simulink model "DrivetrainHevP4"  (R2023b)
settings: Solver=VariableStepAuto  StartTime=0.0  StopTime=inf  RelTol=1e-3  EnableMultiTasking=on
model workspace (MAT data in the model file):
  Aeff = Simulink.Parameter
  Aeff.Value = 0.0314159265359
  Aeff.DataType = 'double'
  Aeff.Complexity = 'real'
  Aeff.Dimensions = [1 1]
  Af = Simulink.Parameter
  Af.Value = 2.46
  Af.DataType = 'double'
  Af.Complexity = 'real'
  Af.Dimensions = [1 1]
  Bx = Simulink.Parameter
  Bx.Value = 10
  Bx.DataType = 'double'
  Bx.Complexity = 'real'
  Bx.Dimensions = [1 1]
  Cd = Simulink.Parameter
  Cd.Value = 0.25
  Cd.DataType = 'double'
  Cd.Complexity = 'real'
  Cd.Dimensions = [1 1]
  Cl = Simulink.Parameter
  Cl.Value = 0.1
  Cl.DataType = 'double'
  Cl.Complexity = 'real'
  Cl.Dimensions = [1 1]
  Cpm = Simulink.Parameter
  Cpm.Value = 0.1
  Cpm.DataType = 'double'
  Cpm.Complexity = 'real'
  Cpm.Dimensions = [1 1]
  Cx = Simulink.Parameter
  Cx.Value = 1.65
  Cx.DataType = 'double'
  Cx.Complexity = 'real'
  Cx.Dimensions = [1 1]
  Dx = Simulink.Parameter
  Dx.Value = 1
  Dx.DataType = 'double'
  Dx.Complexity = 'real'
  Dx.Dimensions = [1 1]
  Ex = Simulink.Parameter
  Ex.Value = 0.01
  Ex.DataType = 'double'
  Ex.Complexity = 'real'
  Ex.Dimensions = [1 1]
  FZMAX = Simulink.Parameter
  FZMAX.Value = 6570
  FZMAX.DataType = 'double'
  FZMAX.Complexity = 'real'
  FZMAX.Dimensions = [1 1]
  FZMIN = Simulink.Parameter
  FZMIN.Value = 0
  FZMIN.DataType = 'double'
  FZMIN.Complexity = 'real'
  FZMIN.Dimensions = [1 1]
  Fc = Simulink.Parameter
  Fc.Value = 500
  Fc.DataType = 'double'
  Fc.Complexity = 'real'
  Fc.Dimensions = [1 1]
  FsbF = Simulink.Parameter
  FsbF.Value = [-700000 -7000 -700 0 700 7000 700000]
  FsbF.DataType = 'double'
  FsbF.Complexity = 'real'
  FsbF.Dimensions = [1 7]
  FsbR = Simulink.Parameter
  FsbR.Value = [-700000 -7000 -700 0 700 7000 700000]
  FsbR.DataType = 'double'
  FsbR.Complexity = 'real'
  FsbR.Dimensions = [1 7]
  FskF = Simulink.Parameter
  FskF.Value = [-8928.57142857 -178.571428571 0 357.142857143 535.714285714 9285.71428571]
  FskF.DataType = 'double'
  FskF.Complexity = 'real'
  FskF.Dimensions = [1 6]
  FskR = Simulink.Parameter
  FskR.Value = [-5357.14285714 -107.142857143 0 214.285714286 321.428571429 5571.42857143]
  FskR.DataType = 'double'
  FskR.Complexity = 'real'
  FskR.Dimensions = [1 6]
  G = Simulink.Parameter
  G.Value = [0 1 2 3 4 5 6]
  G.DataType = 'double'
  G.Complexity = 'real'
  G.Dimensions = [1 7]
  G_o = Simulink.Parameter
  G_o.Value = 1
  G_o.DataType = 'double'
  G_o.Complexity = 'real'
  G_o.Dimensions = [1 1]
  Iyy = Simulink.Parameter
  Iyy.Value = 3000
  Iyy.DataType = 'double'
  Iyy.Complexity = 'real'
  Iyy.Dimensions = [1 1]
  Iyy_Whl = Simulink.Parameter
  Iyy_Whl.Value = 0.8
  Iyy_Whl.DataType = 'double'
  Iyy_Whl.Complexity = 'real'
  Iyy_Whl.Dimensions = [1 1]
  J = Simulink.Parameter
  J.Value = 0.01
  J.DataType = 'double'
  J.Complexity = 'real'
  J.Dimensions = [1 1]
  J1 = Simulink.Parameter
  J1.Value = 0.01
  J1.DataType = 'double'
  J1.Complexity = 'real'
  J1.Dimensions = [1 1]
  J2 = Simulink.Parameter
  J2.Value = 0.01
  J2.DataType = 'double'
  J2.Complexity = 'real'
  J2.Dimensions = [1 1]
  Jd = Simulink.Parameter
  Jd.Value = 0.01
  Jd.DataType = 'double'
  Jd.Complexity = 'real'
  Jd.Dimensions = [1 1]
  Ji = Simulink.Parameter
  Ji.Value = 0.2
  Ji.DataType = 'double'
  Ji.Complexity = 'real'
  Ji.Dimensions = [1 1]
  Jin = Simulink.Parameter
  Jin.Value = 0.05
  Jin.DataType = 'double'
  Jin.Complexity = 'real'
  Jin.Dimensions = [1 1]
  Jin_Cltch = Simulink.Parameter
  Jin_Cltch.Value = 0.2
  Jin_Cltch.DataType = 'double'
  Jin_Cltch.Complexity = 'real'
  Jin_Cltch.Dimensions = [1 1]
  Jin_Cltch2 = Simulink.Parameter
  Jin_Cltch2.Value = 0.01
  Jin_Cltch2.DataType = 'double'
  Jin_Cltch2.Complexity = 'real'
  Jin_Cltch2.Dimensions = [1 1]
  Jout = Simulink.Parameter
  Jout.Value = [0.009 0.01 0.01 0.01 0.01 0.01 0.01]
  Jout.DataType = 'double'
  Jout.Complexity = 'real'
  Jout.Dimensions = [1 7]
  Jout_Cltch = Simulink.Parameter
  Jout_Cltch.Value = 0.01
  Jout_Cltch.DataType = 'double'
  Jout_Cltch.Complexity = 'real'
  Jout_Cltch.Dimensions = [1 1]
  Jout_Cltch2 = Simulink.Parameter
  Jout_Cltch2.Value = 0.05
  Jout_Cltch2.DataType = 'double'
  Jout_Cltch2.Complexity = 'real'
  Jout_Cltch2.Dimensions = [1 1]
  Jt = Simulink.Parameter
  Jt.Value = 0.01
  Jt.DataType = 'double'
  Jt.Complexity = 'real'
  Jt.Dimensions = [1 1]
  Jw1 = Simulink.Parameter
  Jw1.Value = 0.01
  Jw1.DataType = 'double'
  Jw1.Complexity = 'real'
  Jw1.Dimensions = [1 1]
  Jw2 = Simulink.Parameter
  Jw2.Value = 0.01
  Jw2.DataType = 'double'
  Jw2.Complexity = 'real'
  Jw2.Dimensions = [1 1]
  K_c = Simulink.Parameter
  K_c.Value = 10000
  K_c.DataType = 'double'
  K_c.Complexity = 'real'
  K_c.Dimensions = [1 1]
  Lrel = Simulink.Parameter
  Lrel.Value = 0.15
  Lrel.DataType = 'double'
  Lrel.Complexity = 'real'
  Lrel.Dimensions = [1 1]
  Mass = Simulink.Parameter
  Mass.Value = 1623
  Mass.DataType = 'double'
  Mass.Complexity = 'real'
  Mass.Dimensions = [1 1]
  N = Simulink.Parameter
  N.Value = [1 4.212 2.637 1.8 1.386 1 0.772]
  N.DataType = 'double'
  N.Complexity = 'real'
  N.Dimensions = [1 7]
  NF = Simulink.Parameter
  NF.Value = 2
  NF.DataType = 'double'
  NF.Complexity = 'real'
  NF.Dimensions = [1 1]
  NR = Simulink.Parameter
  NR.Value = 2
  NR.DataType = 'double'
  NR.Complexity = 'real'
  NR.Dimensions = [1 1]
  N_P4 = Simulink.Parameter
  N_P4.Value = 4.1
  N_P4.DataType = 'double'
  N_P4.Complexity = 'real'
  N_P4.Dimensions = [1 1]
  Ndiff = Simulink.Parameter
  Ndiff.Value = 3.32
  Ndiff.DataType = 'double'
  Ndiff.Complexity = 'real'
  Ndiff.Dimensions = [1 1]
  Ndiff_P4 = Simulink.Parameter
  Ndiff_P4.Value = 4.1
  Ndiff_P4.DataType = 'double'
  Ndiff_P4.Complexity = 'real'
  Ndiff_P4.Dimensions = [1 1]
  Ndisk = Simulink.Parameter
  Ndisk.Value = 1
  Ndisk.DataType = 'double'
  Ndisk.Complexity = 'real'
  Ndisk.Dimensions = [1 1]
  Ndisks = Simulink.Parameter
  Ndisks.Value = 4
  Ndisks.DataType = 'double'
  Ndisks.Complexity = 'real'
  Ndisks.Dimensions = [1 1]
  Pabs = Simulink.Parameter
  Pabs.Value = 101325
  Pabs.DataType = 'double'
  Pabs.Complexity = 'real'
  Pabs.Dimensions = [1 1]
  Press = Simulink.Parameter
  Press.Value = 7000000
  Press.DataType = 'double'
  Press.Complexity = 'real'
  Press.Dimensions = [1 1]
  Re = Simulink.Parameter
  Re.Value = 0.327
  Re.DataType = 'double'
  Re.Complexity = 'real'
  Re.Dimensions = [1 1]
  Reff = Simulink.Parameter
  Reff.Value = 0.11
  Reff.DataType = 'double'
  Reff.Complexity = 'real'
  Reff.Dimensions = [1 1]
  Reff_LSD = Simulink.Parameter
  Reff_LSD.Value = 0.2
  Reff_LSD.DataType = 'double'
  Reff_LSD.Complexity = 'real'
  Reff_LSD.Dimensions = [1 1]
  Rm = Simulink.Parameter
  Rm.Value = 0.15
  Rm.DataType = 'double'
  Rm.Complexity = 'real'
  Rm.Dimensions = [1 1]
  T = Simulink.Parameter
  T.Value = 300
  T.DataType = 'double'
  T.Complexity = 'real'
  T.Dimensions = [1 1]
  Temp_bpts = Simulink.Parameter
  Temp_bpts.Value = [313 358]
  Temp_bpts.DataType = 'double'
  Temp_bpts.Complexity = 'real'
  Temp_bpts.Dimensions = [1 2]
  Trq_bpts = Simulink.Parameter
  Trq_bpts.Value = [25 50 75 100 150 200 250]
  Trq_bpts.DataType = 'double'
  Trq_bpts.Complexity = 'real'
  Trq_bpts.Dimensions = [1 7]
  UNLOADED_RADIUS = Simulink.Parameter
  UNLOADED_RADIUS.Value = 0.336
  UNLOADED_RADIUS.DataType = 'double'
  UNLOADED_RADIUS.Complexity = 'real'
  UNLOADED_RADIUS.Dimensions = [1 1]
  VXLOW = Simulink.Parameter
  VXLOW.Value = 2
  VXLOW.DataType = 'double'
  VXLOW.Complexity = 'real'
  VXLOW.Dimensions = [1 1]
  aMy = Simulink.Parameter
  aMy.Value = 0.01
  aMy.DataType = 'double'
  aMy.Complexity = 'real'
  aMy.Dimensions = [1 1]
  a_CG = Simulink.Parameter
  a_CG.Value = 1.09
  a_CG.DataType = 'double'
  a_CG.Complexity = 'real'
  a_CG.Dimensions = [1 1]
  alphaMy = Simulink.Parameter
  alphaMy.Value = 0
  alphaMy.DataType = 'double'
  alphaMy.Complexity = 'real'
  alphaMy.Dimensions = [1 1]
  b = Simulink.Parameter
  b.Value = 400
  b.DataType = 'auto'
  b.Complexity = 'real'
  b.Dimensions = [1 1]
  b1 = Simulink.Parameter
  b1.Value = 100
  b1.DataType = 'double'
  b1.Complexity = 'real'
  b1.Dimensions = [1 1]
  b1_g = Simulink.Parameter
  b1_g.Value = 0.001
  b1_g.DataType = 'double'
  b1_g.Complexity = 'real'
  b1_g.Dimensions = [1 1]
  b2 = Simulink.Parameter
  b2.Value = 100
  b2.DataType = 'double'
  b2.Complexity = 'real'
  b2.Dimensions = [1 1]
  b2_g = Simulink.Parameter
  b2_g.Value = 0.001
  b2_g.DataType = 'double'
  b2_g.Complexity = 'real'
  b2_g.Dimensions = [1 1]
  bMy = Simulink.Parameter
  bMy.Value = 0
  bMy.DataType = 'double'
  bMy.Complexity = 'real'
  bMy.Dimensions = [1 1]
  b_CG = Simulink.Parameter
  b_CG.Value = 1.7
  b_CG.DataType = 'double'
  b_CG.Complexity = 'real'
  b_CG.Dimensions = [1 1]
  b_J = Simulink.Parameter
  b_J.Value = 0.001
  b_J.DataType = 'double'
  b_J.Complexity = 'real'
  b_J.Dimensions = [1 1]
  bd = Simulink.Parameter
  bd.Value = 0.001
  bd.DataType = 'double'
  bd.Complexity = 'real'
  bd.Dimensions = [1 1]
  betaMy = Simulink.Parameter
  betaMy.Value = 1
  betaMy.DataType = 'double'
  betaMy.Complexity = 'real'
  betaMy.Dimensions = [1 1]
  bi = Simulink.Parameter
  bi.Value = 0.001
  bi.DataType = 'double'
  bi.Complexity = 'real'
  bi.Dimensions = [1 1]
  bin = Simulink.Parameter
  bin.Value = 0.003
  bin.DataType = 'double'
  bin.Complexity = 'real'
  bin.Dimensions = [1 1]
  bin_Cltch = Simulink.Parameter
  bin_Cltch.Value = 0.003
  bin_Cltch.DataType = 'double'
  bin_Cltch.Complexity = 'real'
  bin_Cltch.Dimensions = [1 1]
  bout = Simulink.Parameter
  bout.Value = [0.003 0.003 0.003 0.003 0.003 0.003 0.003]
  bout.DataType = 'double'
  bout.Complexity = 'real'
  bout.Dimensions = [1 7]
  bout_Cltch = Simulink.Parameter
  bout_Cltch.Value = 0.003
  bout_Cltch.DataType = 'double'
  bout_Cltch.Complexity = 'real'
  bout_Cltch.Dimensions = [1 1]
  br = Simulink.Parameter
  br.Value = 0.001
  br.DataType = 'double'
  br.Complexity = 'real'
  br.Dimensions = [1 1]
  bt = Simulink.Parameter
  bt.Value = 0.001
  bt.DataType = 'double'
  bt.Complexity = 'real'
  bt.Dimensions = [1 1]
  bw1 = Simulink.Parameter
  bw1.Value = 0.001
  bw1.DataType = 'double'
  bw1.Complexity = 'real'
  bw1.Dimensions = [1 1]
  bw2 = Simulink.Parameter
  bw2.Value = 0.001
  bw2.DataType = 'double'
  bw2.Complexity = 'real'
  bw2.Dimensions = [1 1]
  cMy = Simulink.Parameter
  cMy.Value = 0
  cMy.DataType = 'double'
  cMy.Complexity = 'real'
  cMy.Dimensions = [1 1]
  disk_abore = Simulink.Parameter
  disk_abore.Value = 0.05
  disk_abore.DataType = 'double'
  disk_abore.Complexity = 'real'
  disk_abore.Dimensions = [1 1]
  domega_o = Simulink.Parameter
  domega_o.Value = 0
  domega_o.DataType = 'double'
  domega_o.Complexity = 'real'
  domega_o.Dimensions = [1 1]
  dw = Simulink.Parameter
  dw.Value = [0 10 20 40 60 80 100]
  dw.DataType = 'double'
  dw.Complexity = 'real'
  dw.Dimensions = [1 7]
  dzdotsF = Simulink.Parameter
  dzdotsF.Value = [-10 -1 -0.1 0 0.1 1 10]
  dzdotsF.DataType = 'double'
  dzdotsF.Complexity = 'real'
  dzdotsF.Dimensions = [1 7]
  dzdotsR = Simulink.Parameter
  dzdotsR.Value = [-10 -1 -0.1 0 0.1 1 10]
  dzdotsR.DataType = 'double'
  dzdotsR.Complexity = 'real'
  dzdotsR.Dimensions = [1 7]
  dzsF = Simulink.Parameter
  dzsF.Value = [-0.005 -0.0001 0 0.2 0.2001 0.2051]
  dzsF.DataType = 'double'
  dzsF.Complexity = 'real'
  dzsF.Dimensions = [1 6]
  dzsR = Simulink.Parameter
  dzsR.Value = [-0.005 -0.0001 0 0.2 0.2001 0.2051]
  dzsR.DataType = 'double'
  dzsR.Complexity = 'real'
  dzsR.Dimensions = [1 6]
  eta = Simulink.Parameter
  eta.Value = [0.95 0.95 0.95 0.95 0.95 0.95 0.95]
  eta.DataType = 'double'
  eta.Complexity = 'real'
  eta.Dimensions = [1 7]
  eta_diff = Simulink.Parameter
  eta_diff.Value = 0.98
  eta_diff.DataType = 'double'
  eta_diff.Complexity = 'real'
  eta_diff.Dimensions = [1 1]
  eta_tbl = Simulink.Parameter
  eta_tbl.Value = [0.766 0.766 0.766 0.766 0.766 0.766 0.766 0.766 0.766 0.766 0.766 0.766 ... (1078 elements, 7x11x7x2)]
  eta_tbl.DataType = 'double'
  eta_tbl.Complexity = 'real'
  eta_tbl.Dimensions = [7 11 7 2]
  g = Simulink.Parameter
  g.Value = 9.81
  g.DataType = 'double'
  g.Complexity = 'real'
  g.Dimensions = [1 1]
  grEff = Simulink.Parameter
  grEff.Value = [0.766 0.4596 0.504 0.98119 0.917 0.9224 0.9124]
  grEff.DataType = 'double'
  grEff.Complexity = 'real'
  grEff.Dimensions = [1 7]
  h = Simulink.Parameter
  h.Value = 0.5
  h.DataType = 'double'
  h.Complexity = 'real'
  h.Dimensions = [1 1]
  k = Simulink.Parameter
  k.Value = 10000
  k.DataType = 'auto'
  k.Complexity = 'real'
  k.Dimensions = [1 1]
  k1 = Simulink.Parameter
  k1.Value = 50000
  k1.DataType = 'double'
  k1.Complexity = 'real'
  k1.Dimensions = [1 1]
  k2 = Simulink.Parameter
  k2.Value = 50000
  k2.DataType = 'double'
  k2.Complexity = 'real'
  k2.Dimensions = [1 1]
  kappamax = Simulink.Parameter
  kappamax.Value = 1.5
  kappamax.DataType = 'double'
  kappamax.Complexity = 'real'
  kappamax.Dimensions = [1 1]
  lam_x = Simulink.Parameter
  lam_x.Value = 1
  lam_x.DataType = 'double'
  lam_x.Complexity = 'real'
  lam_x.Dimensions = [1 1]
  mu_kinetic = Simulink.Parameter
  mu_kinetic.Value = 0.35
  mu_kinetic.DataType = 'double'
  mu_kinetic.Complexity = 'real'
  mu_kinetic.Dimensions = [1 1]
  mu_static = Simulink.Parameter
  mu_static.Value = 0.45
  mu_static.DataType = 'double'
  mu_static.Complexity = 'real'
  mu_static.Dimensions = [1 1]
  muc = Simulink.Parameter
  muc.Value = [0.16 0.13 0.115 0.11 0.105 0.1025 0.10125]
  muc.DataType = 'double'
  muc.Complexity = 'real'
  muc.Dimensions = [1 7]
  muk = Simulink.Parameter
  muk.Value = 0.4
  muk.DataType = 'double'
  muk.Complexity = 'real'
  muk.Dimensions = [1 1]
  mus = Simulink.Parameter
  mus.Value = 0.45
  mus.DataType = 'double'
  mus.Complexity = 'real'
  mus.Dimensions = [1 1]
  num_pads = Simulink.Parameter
  num_pads.Value = 2
  num_pads.DataType = 'double'
  num_pads.Complexity = 'real'
  num_pads.Dimensions = [1 1]
  omega1_c = Simulink.Parameter
  omega1_c.Value = 3000
  omega1_c.DataType = 'double'
  omega1_c.Complexity = 'real'
  omega1_c.Dimensions = [1 1]
  omega2_c = Simulink.Parameter
  omega2_c.Value = 3000
  omega2_c.DataType = 'double'
  omega2_c.Complexity = 'real'
  omega2_c.Dimensions = [1 1]
  omega_bpts = Simulink.Parameter
  omega_bpts.Value = [500.383141081 749.619781963 1002.67614148 1250.9578527 1499.23956393 1747.52127515 1995.80298637 2501.9157054 2998.47912785 4001.15526933 5003.83141081]
  omega_bpts.DataType = 'double'
  omega_bpts.Complexity = 'real'
  omega_bpts.Dimensions = [1 11]
  omega_c = Simulink.Parameter
  omega_c.Value = 500
  omega_c.DataType = 'auto'
  omega_c.Complexity = 'real'
  omega_c.Dimensions = [1 1]
  omega_o = Simulink.Parameter
  omega_o.Value = 0
  omega_o.DataType = 'double'
  omega_o.Complexity = 'real'
  omega_o.Dimensions = [1 1]
  omega_o_J = Simulink.Parameter
  omega_o_J.Value = 0
  omega_o_J.DataType = 'double'
  omega_o_J.Complexity = 'real'
  omega_o_J.Dimensions = [1 1]
  omegai_o = Simulink.Parameter
  omegai_o.Value = 0
  omegai_o.DataType = 'double'
  omegai_o.Complexity = 'real'
  omegai_o.Dimensions = [1 1]
  omegain_o = Simulink.Parameter
  omegain_o.Value = 0
  omegain_o.DataType = 'double'
  omegain_o.Complexity = 'real'
  omegain_o.Dimensions = [1 1]
  omegal = Simulink.Parameter
  omegal.Value = 94.2477796077
  omegal.DataType = 'double'
  omegal.Complexity = 'real'
  omegal.Dimensions = [1 1]
  omegao = Simulink.Parameter
  omegao.Value = 0
  omegao.DataType = 'double'
  omegao.Complexity = 'real'
  omegao.Dimensions = [1 1]
  omegaout_o = Simulink.Parameter
  omegaout_o.Value = 0
  omegaout_o.DataType = 'double'
  omegaout_o.Complexity = 'real'
  omegaout_o.Dimensions = [1 1]
  omegat_o = Simulink.Parameter
  omegat_o.Value = 0
  omegat_o.DataType = 'double'
  omegat_o.Complexity = 'real'
  omegat_o.Dimensions = [1 1]
  omegau = Simulink.Parameter
  omegau.Value = 83.7758040957
  omegau.DataType = 'double'
  omegau.Complexity = 'real'
  omegau.Dimensions = [1 1]
  omegaw1o = Simulink.Parameter
  omegaw1o.Value = 0
  omegaw1o.DataType = 'double'
  omegaw1o.Complexity = 'real'
  omegaw1o.Dimensions = [1 1]
  omegaw2o = Simulink.Parameter
  omegaw2o.Value = 0
  omegaw2o.DataType = 'double'
  omegaw2o.Complexity = 'real'
  omegaw2o.Dimensions = [1 1]
  phi = Simulink.Parameter
  phi.Value = [0 0.5 0.6 0.7 0.8 0.87 0.92 0.94 0.96 0.97]
  phi.DataType = 'double'
  phi.Complexity = 'real'
  phi.Dimensions = [1 10]
  philu = Simulink.Parameter
  philu.Value = 0.85
  philu.DataType = 'double'
  philu.Complexity = 'real'
  philu.Dimensions = [1 1]
  press = Simulink.Parameter
  press.Value = 234400
  press.DataType = 'double'
  press.Complexity = 'real'
  press.Dimensions = [1 1]
  psi = Simulink.Parameter
  psi.Value = [12.2938 12.8588 13.1452 13.6285 14.6163 16.2675 19.3503 22.1046 29.9986 50]
  psi.DataType = 'double'
  psi.Complexity = 'real'
  psi.Dimensions = [1 10]
  q_o = Simulink.Parameter
  q_o.Value = 0
  q_o.DataType = 'double'
  q_o.Complexity = 'real'
  q_o.Dimensions = [1 1]
  tauC = Simulink.Parameter
  tauC.Value = 0.6
  tauC.DataType = 'double'
  tauC.Complexity = 'real'
  tauC.Dimensions = [1 1]
  tauC_1 = Simulink.Parameter
  tauC_1.Value = 0.1
  tauC_1.DataType = 'double'
  tauC_1.Complexity = 'real'
  tauC_1.Dimensions = [1 1]
  tauC_LSD = Simulink.Parameter
  tauC_LSD.Value = 0.01
  tauC_LSD.DataType = 'double'
  tauC_LSD.Complexity = 'real'
  tauC_LSD.Dimensions = [1 1]
  tauTC = Simulink.Parameter
  tauTC.Value = 0.1
  tauTC.DataType = 'double'
  tauTC.Complexity = 'real'
  tauTC.Dimensions = [1 1]
  tau_s = Simulink.Parameter
  tau_s.Value = 0.08
  tau_s.DataType = 'double'
  tau_s.Complexity = 'real'
  tau_s.Dimensions = [1 1]
  tc = Simulink.Parameter
  tc.Value = 0.01
  tc.DataType = 'double'
  tc.Complexity = 'real'
  tc.Dimensions = [1 1]
  theta_o = Simulink.Parameter
  theta_o.Value = 0
  theta_o.DataType = 'double'
  theta_o.Complexity = 'real'
  theta_o.Dimensions = [1 1]
  theta_o_Veh = Simulink.Parameter
  theta_o_Veh.Value = 0
  theta_o_Veh.DataType = 'double'
  theta_o_Veh.Complexity = 'real'
  theta_o_Veh.Dimensions = [1 1]
  ts = Simulink.Parameter
  ts.Value = 0.01
  ts.DataType = 'double'
  ts.Complexity = 'real'
  ts.Dimensions = [1 1]
  w1_o = Simulink.Parameter
  w1_o.Value = 0
  w1_o.DataType = 'double'
  w1_o.Complexity = 'real'
  w1_o.Dimensions = [1 1]
  wc = Simulink.Parameter
  wc.Value = 10
  wc.DataType = 'double'
  wc.Complexity = 'real'
  wc.Dimensions = [1 1]
  win_o = Simulink.Parameter
  win_o.Value = 0
  win_o.DataType = 'double'
  win_o.Complexity = 'real'
  win_o.Dimensions = [1 1]
  wout_o = Simulink.Parameter
  wout_o.Value = 0
  wout_o.DataType = 'double'
  wout_o.Complexity = 'real'
  wout_o.Dimensions = [1 1]
  x_o = Simulink.Parameter
  x_o.Value = 0
  x_o.DataType = 'double'
  x_o.Complexity = 'real'
  x_o.Dimensions = [1 1]
  xdot_o = Simulink.Parameter
  xdot_o.Value = 0
  xdot_o.DataType = 'double'
  xdot_o.Complexity = 'real'
  xdot_o.Dimensions = [1 1]
  z_o = Simulink.Parameter
  z_o.Value = -0.35
  z_o.DataType = 'double'
  z_o.Complexity = 'real'
  z_o.Dimensions = [1 1]
  zdot_o = Simulink.Parameter
  zdot_o.Value = 0
  zdot_o.DataType = 'double'
  zdot_o.Complexity = 'real'
  zdot_o.Dimensions = [1 1]
  zeta = Simulink.Parameter
  zeta.Value = [2.232 1.5462 1.4058 1.2746 1.1528 1.0732 1.0192 0.9983 0.9983 0.9983]
  zeta.DataType = 'double'
  zeta.Complexity = 'real'
  zeta.Dimensions = [1 10]
undefined symbols (not defined in the file or in its folder): Lock, up
libraries: autolibsharedcoupling x4, autolibpowerinfoutils x4, autolibshared x3, autolibshareddiff x2, autolibutils x2, autolibsharedtransfixedgear x1, autolibtrqconv x1
(part 1 of 3)
settings Model: DataDictionary=DrivetrainHevP4.sldd  EnableAccessToBaseWorkspace=off  ModifiedByFormat=The MathWorks, Inc.  SimulationMode=accelerator  PauseTimes=10  Creator=The MathWorks, Inc.  LastModifiedBy=The MathWorks, Inc.
settings SolverCC: AlgebraicLoopSolver=TrustRegion  DecoupledContinuousIntegration=on  MaxZcPerStep=1
settings DataIOCC: DSMLogging=off  ReturnWorkspaceOutputs=off
settings DebuggingCC: MergeDetectMultiDrivingBlocksExec=none  UnconnectedInputMsg=warning  UnconnectedOutputMsg=warning  UnconnectedLineMsg=warning  SubsystemReferenceDiagnosticForUnitTest=warning  ArithmeticOperatorsInVariantConditions=warning
settings ModelReferenceCC: EnableRefExpFcnMdlSchedulingChecks=on  PropagateSignalLabelsOutOfModel=off
settings SFSimCC: SimUseLocalCustomCode=off
settings RTWCC: RTWUseLocalCustomCode=off  DLArmComputeVersion=19.05
settings CodeAppCC: StateflowObjectComments=on
settings GRTTargetCC: TargetLangStandard=C89/C90 (ANSI)
settings ConfigComp: CovMetricSettings=dsw  CovSaveCumulativeToWorkspaceVar=on  CovSaveSingleToWorkspaceVar=on  CovExternalEMLEnable=off
settings SimscapeCC: SimscapeNormalizeSystem=off  SimscapeNominalValues={1, 'bar'; 1, 'cm^3/s'; 1, 'bar*kg/s'; 1, 'kJ/kg'; 1, 'kW'; }

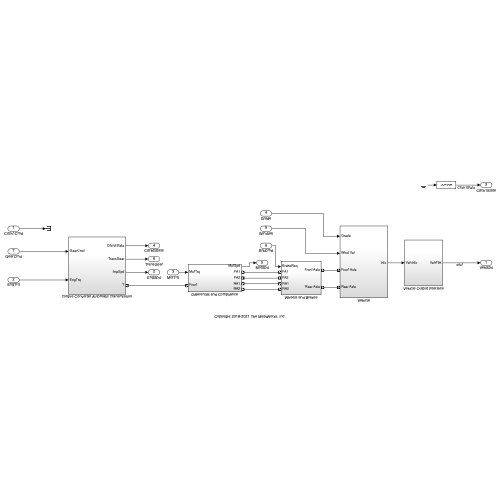
[thumbnail: Simulink's stored preview of the top-level diagram]
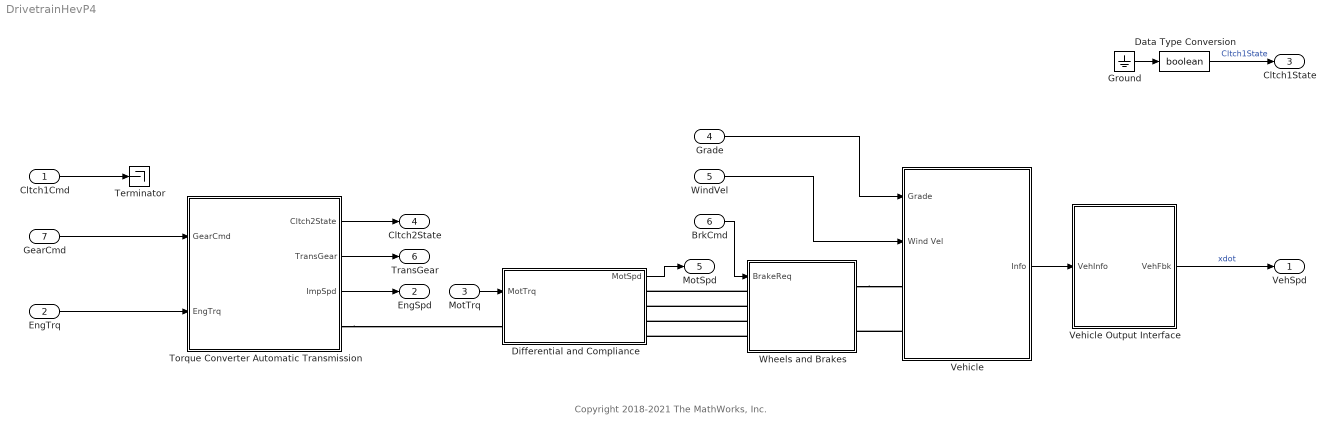
== system DrivetrainHevP4 ==
  note: Copyright 2018-2021 The MathWorks, Inc.
  Cltch1Cmd : Inport
  EngTrq : Inport  Port=2
  MotTrq : Inport  Port=3
  Grade : Inport  Port=4
  WindVel : Inport  Port=5
  BrkCmd : Inport  Port=6
  GearCmd : Inport  Port=7
  Data Type Conversion : DataTypeConversion  OutDataTypeStr=boolean  SaturateOnIntegerOverflow=off  RndMeth=Floor
  Differential and Compliance : Subsystem  VariantControl=2
  Ground : Ground
  Terminator : Terminator
  Torque Converter Automatic Transmission : Subsystem  VariantControl=1
  Vehicle : Subsystem
  Vehicle Output Interface : Subsystem
  Wheels and Brakes : Subsystem  VariantControl=0
  VehSpd : Outport  VectorParamsAs1DForOutWhenUnconnected=off
  EngSpd : Outport  Port=2  VectorParamsAs1DForOutWhenUnconnected=off  BusOutputAsStruct=on
  Cltch1State : Outport  Port=3  VectorParamsAs1DForOutWhenUnconnected=off  BusOutputAsStruct=on
  Cltch2State : Outport  Port=4  VectorParamsAs1DForOutWhenUnconnected=off  BusOutputAsStruct=on
  MotSpd : Outport  Port=5  VectorParamsAs1DForOutWhenUnconnected=off  BusOutputAsStruct=on
  TransGear : Outport  Port=6  VectorParamsAs1DForOutWhenUnconnected=off  BusOutputAsStruct=on
  wires:
  BrkCmd/1 -> Wheels and Brakes/1(BrakeReq)
  Vehicle/1(Info) -> Vehicle Output Interface/1(VehInfo)
  Vehicle Output Interface/1(VehFbk) -> VehSpd/1  "xdot"
  Grade/1 -> Vehicle/1(Grade)
  WindVel/1 -> Vehicle/2(Wind Vel)
  Ground/1 -> Data Type Conversion/1
  Data Type Conversion/1 -> Cltch1State/1  "Cltch1State"
  Torque Converter Automatic Transmission/1(Cltch2State) -> Cltch2State/1
  Torque Converter Automatic Transmission/2(TransGear) -> TransGear/1
  Cltch1Cmd/1 -> Terminator/1
  GearCmd/1 -> Torque Converter Automatic Transmission/1(GearCmd)
  MotTrq/1 -> Differential and Compliance/1(MotTrq)
  EngTrq/1 -> Torque Converter Automatic Transmission/2(EngTrq)
  Torque Converter Automatic Transmission/3(ImpSpd) -> EngSpd/1
  Differential and Compliance/1(MotSpd) -> MotSpd/1
  connections:
  Wheels and Brakes/RConn1 -- Vehicle/LConn1
  Wheels and Brakes/LConn1 -- Differential and Compliance/RConn1
  Wheels and Brakes/LConn3 -- Differential and Compliance/RConn3
  Wheels and Brakes/LConn2 -- Differential and Compliance/RConn2
  Wheels and Brakes/LConn4 -- Differential and Compliance/RConn4
  Vehicle/LConn2 -- Wheels and Brakes/RConn2
  Torque Converter Automatic Transmission/RConn1 -- Differential and Compliance/LConn1

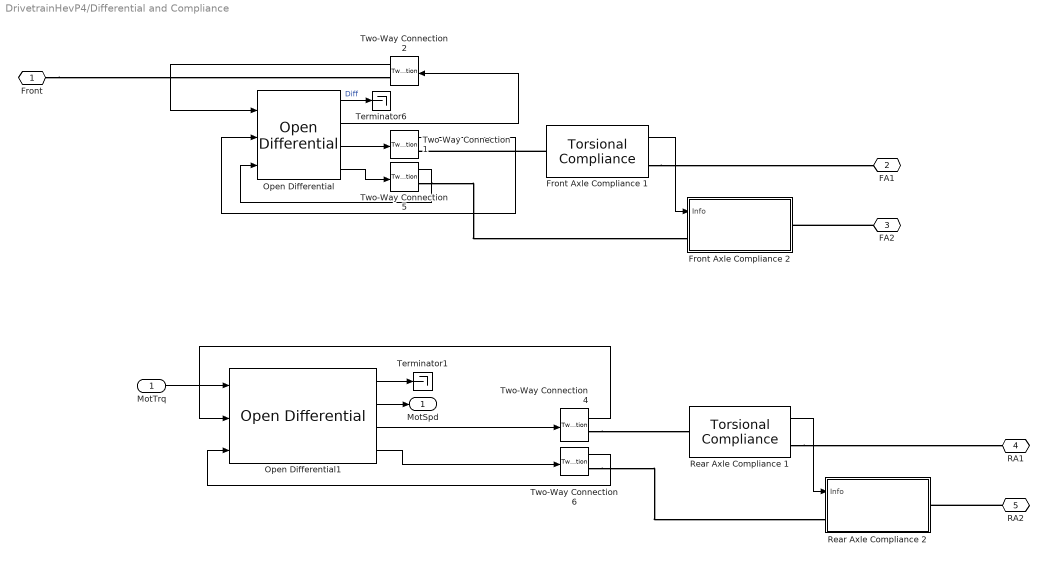
== system DrivetrainHevP4/Differential and Compliance ==
  MotTrq : Inport
  Front Axle Compliance 1 : autolibsharedcoupling/Torsional Compliance  port_config=Two-way connection  extInfo=on  k=k  b=b  theta_o=theta_o  domega_o=domega_o  omega_c=omega_c  blkID=0  aMode=1
  Front Axle Compliance 2 : Subsystem
  Open Differential : autolibshareddiff/Open Differential  DiffEffModelPopup=Constant  InterpMethod=Linear point-slope  extTamb=off  shaftSwitchMask=To the left of center-line  Ndiff=Ndiff  Jd=Jd  bd=bd  Jw1=Jw1  bw1=bw1  Jw2=Jw2  bw2=bw2  omegaw1o=omegaw1o  omegaw2o=omegaw2o  eta=eta_diff  eta_tbl=reshape([0.64 0.76 0.8 0.81 0.83 0.84 0.84 0.56 0.73 0.78 0.8 0.83 0.84 0.84 0.54 0.71 0.77 0.8 0.82 0.84 0.84 0.53 0.71 0.77 0.8 0.83 0.84 0.84 0.51 0.71 0.77 0.8 0.83 0.84 0.85 0.52 0.7 0.77 0.8 0.83 0.84 0.85 0.51 0.71 0.76 0.79 0.83 0.84 0.85 0.5 0.69 0.76 0.79 0.82 0.84 0.85 0.45 0.68 0.75 0.78 0.82 0.84 0.85 0.43 0.67 0.74 0.78 0.81 0.83 0.84 0.38 0.63 0.71 0.75 0.8 0.82 0.83 0.81 0.86 0.88 0.89 0.89 0.89 0.9 0.77 0.85 0.87 0.88 0.89 0.9 0.9 0.72 0.82 0.86 0.87 0.88 0.89 0.9 0.68 0.8 0.84 0.86 0.88 0.89 0.89 0.67 0.8 0.84 0.86 0.88 0.89 0.9 0.67 0.8 0.84 0.86 0.88 0.89 0.9 0.65 0.8 0.84 0.86 0.88 0.89 0.9 0.64 0.79 0.83 0.86 0.88 0.89 0.9 0.63 0.78 0.83 0.86 0.88 0.89 0.9 0.59 0.76 0.82 0.85 0.87 0.89 0.9 0.53 0.73 0.8 0.83 0.86 0.88 0.89], 7, 11, 2)  Trq_bpts=[25, 50, 75, 100, 150, 200, 250]  omega_bpts=[52.4 78.5 105 131 157 183 209 262 314 419 524]  Temp_bpts=[290 358]  Tamb=297.15  maxAbsSpd=5e3  aMode=1
      settings: LibrarySourceBlock=autolibdiff/Open Differential
  Open Differential1 : autolibshareddiff/Open Differential  DiffEffModelPopup=Constant  InterpMethod=Linear point-slope  extTamb=off  shaftSwitchMask=To the left of center-line  Ndiff=Ndiff_P4  Jd=Jd  bd=bd  Jw1=Jw1  bw1=bw1  Jw2=Jw2  bw2=bw2  omegaw1o=omegaw1o  omegaw2o=omegaw2o  eta=eta_diff  eta_tbl=reshape([0.64 0.76 0.8 0.81 0.83 0.84 0.84 0.56 0.73 0.78 0.8 0.83 0.84 0.84 0.54 0.71 0.77 0.8 0.82 0.84 0.84 0.53 0.71 0.77 0.8 0.83 0.84 0.84 0.51 0.71 0.77 0.8 0.83 0.84 0.85 0.52 0.7 0.77 0.8 0.83 0.84 0.85 0.51 0.71 0.76 0.79 0.83 0.84 0.85 0.5 0.69 0.76 0.79 0.82 0.84 0.85 0.45 0.68 0.75 0.78 0.82 0.84 0.85 0.43 0.67 0.74 0.78 0.81 0.83 0.84 0.38 0.63 0.71 0.75 0.8 0.82 0.83 0.81 0.86 0.88 0.89 0.89 0.89 0.9 0.77 0.85 0.87 0.88 0.89 0.9 0.9 0.72 0.82 0.86 0.87 0.88 0.89 0.9 0.68 0.8 0.84 0.86 0.88 0.89 0.89 0.67 0.8 0.84 0.86 0.88 0.89 0.9 0.67 0.8 0.84 0.86 0.88 0.89 0.9 0.65 0.8 0.84 0.86 0.88 0.89 0.9 0.64 0.79 0.83 0.86 0.88 0.89 0.9 0.63 0.78 0.83 0.86 0.88 0.89 0.9 0.59 0.76 0.82 0.85 0.87 0.89 0.9 0.53 0.73 0.8 0.83 0.86 0.88 0.89], 7, 11, 2)  Trq_bpts=[25, 50, 75, 100, 150, 200, 250]  omega_bpts=[52.4 78.5 105 131 157 183 209 262 314 419 524]  Temp_bpts=[290 358]  Tamb=297.15  maxAbsSpd=5e3  aMode=1
      settings: LibrarySourceBlock=autolibdiff/Open Differential
  Rear Axle Compliance 1 : autolibsharedcoupling/Torsional Compliance  port_config=Two-way connection  extInfo=on  k=k  b=b  theta_o=theta_o  domega_o=domega_o  omega_c=omega_c  blkID=0  aMode=1
  Rear Axle Compliance 2 : Subsystem
  Terminator1 : Terminator
  Terminator6 : Terminator
  Two-Way Connection{1..2,4..6} (5 alike) : TwoWayConnection
  Front : PMIOPort  Side=Left
  FA1 : PMIOPort  Port=2  Side=Right
  FA2 : PMIOPort  Port=3  Side=Right
  RA1 : PMIOPort  Port=4  Side=Right
  RA2 : PMIOPort  Port=5  Side=Right
  MotSpd : Outport  VectorParamsAs1DForOutWhenUnconnected=off
  wires:
  Two-Way Connection6/1 -> Open Differential1/3
  Open Differential1/4 -> Two-Way Connection6/1
  Rear Axle Compliance 1/1 -> Rear Axle Compliance 2/1(Info)
  Two-Way Connection5/1 -> Open Differential/3
  Open Differential/4 -> Two-Way Connection5/1
  Front Axle Compliance 1/1 -> Front Axle Compliance 2/1(Info)
  Two-Way Connection4/1 -> Open Differential1/2
  Open Differential1/3 -> Two-Way Connection4/1
  Open Differential1/1 -> Terminator1/1
  Open Differential/2 -> Two-Way Connection2/1
  Open Differential/3 -> Two-Way Connection1/1
  Two-Way Connection1/1 -> Open Differential/2
  Two-Way Connection2/1 -> Open Differential/1
  Open Differential/1 -> Terminator6/1  "Diff"
  Open Differential1/2 -> MotSpd/1
  MotTrq/1 -> Open Differential1/1
  connections:
  Two-Way Connection6/RConn1 -- Rear Axle Compliance 2/LConn1
  Rear Axle Compliance 1/RConn1 -- RA1/RConn1
  Two-Way Connection4/RConn1 -- Rear Axle Compliance 1/LConn1
  RA2/RConn1 -- Rear Axle Compliance 2/RConn1
  Front Axle Compliance 1/LConn1 -- Two-Way Connection1/RConn1
  Front Axle Compliance 1/RConn1 -- FA1/RConn1
  FA2/RConn1 -- Front Axle Compliance 2/RConn1
  Two-Way Connection5/RConn1 -- Front Axle Compliance 2/LConn1
  Front/RConn1 -- Two-Way Connection2/RConn1

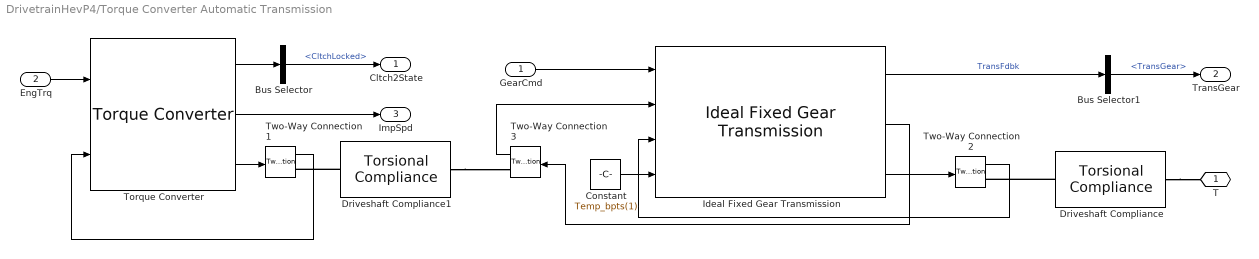
== system DrivetrainHevP4/Torque Converter Automatic Transmission ==
  GearCmd : Inport
  EngTrq : Inport  Port=2
  Bus Selector : BusSelector  OutputSignals=Cltch.CltchLocked
  Bus Selector1 : BusSelector  OutputSignals=Trans.TransGear
  Constant : Constant  Value=Temp_bpts(1)
  Driveshaft Compliance : autolibsharedcoupling/Torsional Compliance  port_config=Two-way connection  extInfo=off  k=k  b=b  theta_o=theta_o  domega_o=domega_o  omega_c=omega_c  blkID=0  aMode=1
  Driveshaft Compliance1 : autolibsharedcoupling/Torsional Compliance  port_config=Two-way connection  extInfo=off  k=k  b=b  theta_o=theta_o  domega_o=domega_o  omega_c=omega_c  blkID=0  aMode=1
  Ideal Fixed Gear Transmission : autolibsharedtransfixedgear/Ideal Fixed Gear Transmission  VariantControl=0  TransEffModelPopup=Gear, input torque, input speed, and temperature  gearInterp=Linear point-slope  G=G  Trq_bpts=Trq_bpts  omega_bpts=omega_bpts  Temp_bpts=Temp_bpts  N=N  Jout=Jout  bout=bout  eta=eta  eta_tbl=eta_tbl  G_o=0  omega_o=omega_o  omegaN_o=0  tau_s=tau_s  maxAbsSpd=5e3  aMode=1
      settings: LibrarySourceBlock=autolibtrans/Ideal Fixed Gear Transmission
  Torque Converter : autolibtrqconv/Torque Converter  TCType=Lock-up  port_config=Simulink  Ji=Ji  bi=bi  Jt=Jt  bt=bt  omegai_o=omegai_o  omegat_o=omegat_o  phi=phi  KType=Input speed / sqrt(input torque)  psi=psi  zeta=zeta  tauTC=tauTC  InterpMethod=Linear  Reff=Reff  mus=mus  muk=muk  ClutchLocked=off  philu=philu  omegal=omegal  omegau=omegau  K_c=K_c  tauC=tauC  maxAbsSpd=5e3  tau_dl=3000
      settings: AttributesFormatString="Lock-up type:  %<TCType>"
  Two-Way Connection1 : TwoWayConnection
  Two-Way Connection2 : TwoWayConnection
  Two-Way Connection3 : TwoWayConnection
  T : PMIOPort  Side=Right
  Cltch2State : Outport  VectorParamsAs1DForOutWhenUnconnected=off
  TransGear : Outport  Port=2  VectorParamsAs1DForOutWhenUnconnected=off
  ImpSpd : Outport  Port=3  VectorParamsAs1DForOutWhenUnconnected=off
  wires:
  Bus Selector1/1 -> TransGear/1  "<TransGear>"
  Constant/1 -> Ideal Fixed Gear Transmission/4
  Bus Selector/1 -> Cltch2State/1  "<CltchLocked>"
  Two-Way Connection3/1 -> Ideal Fixed Gear Transmission/2
  EngTrq/1 -> Torque Converter/1
  Ideal Fixed Gear Transmission/3 -> Two-Way Connection2/1
  Two-Way Connection1/1 -> Torque Converter/2
  Two-Way Connection2/1 -> Ideal Fixed Gear Transmission/3
  Torque Converter/3 -> Two-Way Connection1/1
  Ideal Fixed Gear Transmission/2 -> Two-Way Connection3/1
  Torque Converter/1 -> Bus Selector/1
  Torque Converter/2 -> ImpSpd/1
  Ideal Fixed Gear Transmission/1 -> Bus Selector1/1  "TransFdbk"
  GearCmd/1 -> Ideal Fixed Gear Transmission/1
  connections:
  Driveshaft Compliance/RConn1 -- T/RConn1
  Driveshaft Compliance1/LConn1 -- Two-Way Connection1/RConn1
  Driveshaft Compliance/LConn1 -- Two-Way Connection2/RConn1
  Driveshaft Compliance1/RConn1 -- Two-Way Connection3/RConn1

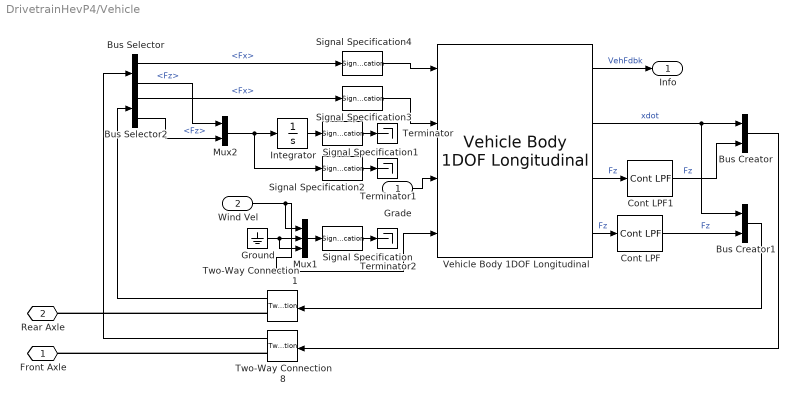
== system DrivetrainHevP4/Vehicle ==
  Grade : Inport  Unit=deg
  Wind Vel : Inport  Port=2  Unit=m/s
  Bus Creator : BusCreator  Inputs=2
  Bus Creator1 : BusCreator  Inputs=2
  Bus Selector : BusSelector  OutputSignals=Fx,Fz
  Bus Selector2 : BusSelector  OutputSignals=Fx,Fz
  Cont LPF : autolibutils/Cont LPF  wc=wc  AbsoluteTolerance=auto  aMode=aMode
  Cont LPF1 : autolibutils/Cont LPF  wc=wc  AbsoluteTolerance=auto  aMode=aMode
  Ground : Ground
  Integrator : Integrator
  Mux1 : Mux  Inputs=3
  Mux2 : Mux  Inputs=2
  Signal Specification : SignalSpecification  Unit=m/s
  Signal Specification1 : SignalSpecification  Unit=m
  Signal Specification2 : SignalSpecification  Unit=m/s
  Signal Specification3 : SignalSpecification  Unit=N
  Signal Specification4 : SignalSpecification  Unit=N
  Terminator : Terminator
  Terminator1 : Terminator
  Terminator2 : Terminator
  Two-Way Connection1 : TwoWayConnection
  Two-Way Connection8 : TwoWayConnection
  Vehicle Body 1DOF Longitudinal : autolibshared/Vehicle Body 1DOF Longitudinal  VariantControl=SL  extFMode=off  extMMode=off  extTamb=off  wind3D=off  aMode=1  NF=NF  NR=NR  m=Mass  a=a_CG  b=b_CG  h=h  Cd=Cd  Cl=0  Cpm=0  Af=Af  x_o=x_o  xdot_o=xdot_o  Pabs=Pabs  T=T  g=g
      settings: LibrarySourceBlock=autolibvehdynlong/Vehicle Body 1DOF Longitudinal
  Front Axle : PMIOPort  Side=Left
  Rear Axle : PMIOPort  Port=2  Side=Left
  Info : Outport  VectorParamsAs1DForOutWhenUnconnected=off
  wires:
  Two-Way Connection1/1 -> Bus Selector2/1
  Bus Selector2/2 -> Mux2/2  "<Fz>"
  Bus Selector2/1 -> Signal Specification3/1  "<Fx>"
  Bus Selector/2 -> Mux2/1  "<Fz>"
  Bus Selector/1 -> Signal Specification4/1  "<Fx>"
  Bus Creator1/1 -> Two-Way Connection1/1
  Bus Creator/1 -> Two-Way Connection8/1
  Signal Specification4/1 -> Vehicle Body 1DOF Longitudinal/1
  Signal Specification3/1 -> Vehicle Body 1DOF Longitudinal/2
  Signal Specification2/1 -> Terminator1/1
  Signal Specification1/1 -> Terminator/1
  Signal Specification/1 -> Terminator2/1
  Grade/1 -> Vehicle Body 1DOF Longitudinal/3
  Wind Vel/1 -> Vehicle Body 1DOF Longitudinal/4, Mux1/1
  Integrator/1 -> Signal Specification1/1
  Mux2/1 -> Signal Specification2/1, Integrator/1
  Vehicle Body 1DOF Longitudinal/4 -> Cont LPF/1  "Fz"
  Mux1/1 -> Signal Specification/1
  Ground/1 -> Mux1/3, Mux1/2
  Vehicle Body 1DOF Longitudinal/1 -> Info/1  "VehFdbk"
  Two-Way Connection8/1 -> Bus Selector/1
  Vehicle Body 1DOF Longitudinal/2 -> Bus Creator/1, Bus Creator1/1  "xdot"
  Vehicle Body 1DOF Longitudinal/3 -> Cont LPF1/1  "Fz"
  Cont LPF/1 -> Bus Creator1/2  "Fz"
  Cont LPF1/1 -> Bus Creator/2  "Fz"
  connections:
  Two-Way Connection1/RConn1 -- Rear Axle/RConn1
  Two-Way Connection8/RConn1 -- Front Axle/RConn1

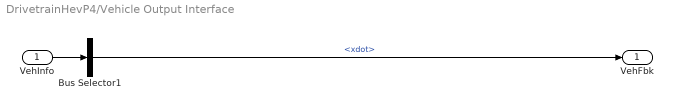
== system DrivetrainHevP4/Vehicle Output Interface ==
  VehInfo : Inport
  Bus Selector1 : BusSelector  OutputSignals=BdyFrm.Cg.Vel.xdot
  VehFbk : Outport  VectorParamsAs1DForOutWhenUnconnected=off
  wires:
  Bus Selector1/1 -> VehFbk/1  "<xdot>"
  VehInfo/1 -> Bus Selector1/1
